simulink model "Magman_LQI"  (R2016b)
settings: Solver=VariableStepAuto  StartTime=0.0  StopTime=35  RelTol=1e-3
values from neighbouring files (symbols this model uses):
  A = [0 1;0 -mu/m]    [PID_script.m]    (also in fminsim.m = []; model_generation.m = [ 0 1 ; 0 0])
  a = 5.713e-09    [LQI_script.m]    (also in PID_script.m = 4.367e-09; fminsim.m = block.InputPort(3).Data; model_generation.m = 4.367e-09)
  b = 0.000324    [LQI_script.m]    (also in PID_script.m = 0.0002827; fminsim.m = block.InputPort(4).Data; model_generation.m = 0.0002827)
  C = [1 0]    [PID_script.m]    (also in model_generation.m)
  D = 0    [PID_script.m]
  h = 0.01    [LQI_script.m]    (also in PID_script.m; model_generation.m)
  K = lqi(sys,q,r,N)    [LQI_script.m]
  linpos = (x2+x3)/2    (= 0.06255)    [LQI_script.m]
  m = 56.3/1000    (= 0.0563)    [LQI_script.m]    (also in PID_script.m; model_generation.m)
  mu = 0.04    [LQI_script.m]    (also in PID_script.m)
  pos_var = 5e-09    [LQI_script.m]    (also in PID_script.m)
  R = pos_var    (= 5e-09)    [LQI_script.m]
  ref = linpos+0.007    (= 0.06955)    [LQI_script.m]
  x00 = linpos-0.013    (= 0.04955)    [LQI_script.m]    (also in PID_script.m = 0.03)
  x1 = 0.02525    [LQI_script.m]    (also in PID_script.m; fminsim.m = block.InputPort(5).Data; model_generation.m)
  x2 = 0.05    [LQI_script.m]    (also in PID_script.m; fminsim.m = block.InputPort(6).Data; model_generation.m)
  x3 = 0.0751    [LQI_script.m]    (also in PID_script.m; fminsim.m = block.InputPort(7).Data; model_generation.m)
  x4 = 0.103    [LQI_script.m]    (also in PID_script.m; fminsim.m = block.InputPort(8).Data; model_generation.m)
undefined symbols (not defined in the file or in its folder): Bkalm, Discrete, Time
libraries: ctrlSharedLib x1, dspsrcs4 x1
settings Model: Creator=Andres  LastModifiedBy=Andres

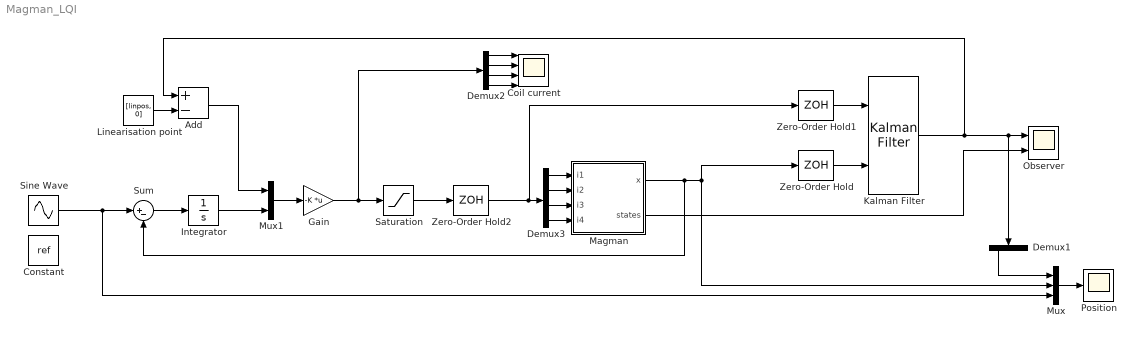
== system Magman_LQI ==
  Add : Sum  Inputs=+-
  Coil current : Scope  NumInputPorts=4
  Constant : Constant  Value=ref
  Demux1 : Demux  Outputs=2
  Demux2 : Demux
  Demux3 : Demux
  Gain : Gain  Gain=-K  Multiplication=Matrix(K*u)
  Integrator : Integrator
  Kalman Filter : ctrlSharedLib/Kalman Filter  TimeDomain=Discrete-Time  UseCurrentEstimator=off  ModelSource=LTI State-Space Variable  ModelSourceVariable=sys_d  A=A  B=Bkalm  C=C  D=D  NumberOfStates=1  NumberOfInputs=1  NumberOfOutputs=1  InitialEstimateSource=Dialog  X0=[0;x00]  P0=10  UseK=off  UseGH=off  NumberOfProcessNoiseInputs=1  G=1  TimeInvariantG=on  H=0  TimeInvariantH=on  Q=Q  TimeInvariantQ=on  R=R  TimeInvariantR=on  N=0  TimeInvariantN=on  AddInputPort=on  AddEnablePort=off  OutputEstimatedY=off  OutputP=off  Ts=-1
  Linearisation point : Constant  Value=[linpos, 0]
  Magman : Subsystem
  Mux : Mux  Inputs=3
  Mux1 : Mux  Inputs=2
  Observer : Scope  NumInputPorts=2
  Position : Scope
  Saturation : Saturate  UpperLimit=0.45  LowerLimit=0
  Sine Wave : Sin  Amplitude=0.005  Bias=x2  Frequency=0.5  SampleTime=0
  Sum : Sum  Inputs=|+-
  Zero-Order Hold : ZeroOrderHold  SampleTime=h
  Zero-Order Hold1 : ZeroOrderHold  SampleTime=h
  Zero-Order Hold2 : ZeroOrderHold  SampleTime=h
  wires:
  Zero-Order Hold2/1 -> Zero-Order Hold1/1, Demux3/1
  Magman/1(x) -> Sum/2, Mux/2, Zero-Order Hold/1
  Kalman Filter/1 -> Demux1/1, Observer/1, Add/1
  Saturation/1 -> Zero-Order Hold2/1
  Demux2/1 -> Coil current/1
  Demux2/2 -> Coil current/2
  Demux2/3 -> Coil current/3
  Demux2/4 -> Coil current/4
  Gain/1 -> Demux2/1, Saturation/1
  Mux1/1 -> Gain/1
  Integrator/1 -> Mux1/2
  Sum/1 -> Integrator/1
  Sine Wave/1 -> Mux/3, Sum/1
  Mux/1 -> Position/1
  Demux3/1 -> Magman/1(i1)
  Demux3/2 -> Magman/2(i2)
  Demux3/3 -> Magman/3(i3)
  Demux3/4 -> Magman/4(i4)
  Zero-Order Hold/1 -> Kalman Filter/2
  Zero-Order Hold1/1 -> Kalman Filter/1
  Demux1/1 -> Mux/1
  Magman/2(states) -> Observer/2
  Linearisation point/1 -> Add/2
  Add/1 -> Mux1/1

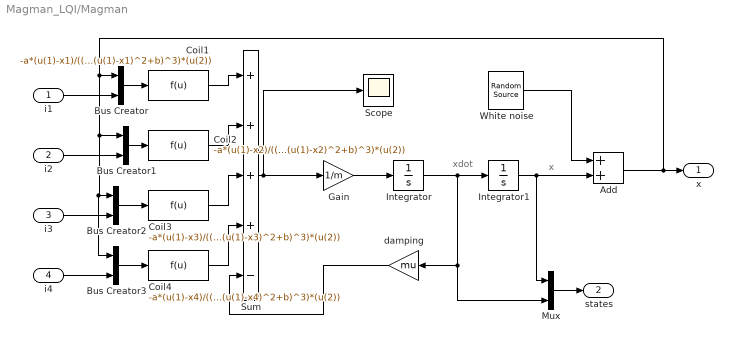
== system Magman_LQI/Magman ==
  note: x
  note: xdot
  i1 : Inport
  i2 : Inport  Port=2
  i3 : Inport  Port=3
  i4 : Inport  Port=4
  Add : Sum
  Bus Creator{,1..3} (4 alike) : BusCreator  Inputs=2
  Coil1 : Fcn  Expr=-a*(u(1)-x1)/(((u(1)-x1)^2+b)^3)*(u(2))
  Coil2 : Fcn  Expr=-a*(u(1)-x2)/(((u(1)-x2)^2+b)^3)*(u(2))
  Coil3 : Fcn  Expr=-a*(u(1)-x3)/(((u(1)-x3)^2+b)^3)*(u(2))
  Coil4 : Fcn  Expr=-a*(u(1)-x4)/(((u(1)-x4)^2+b)^3)*(u(2))
  Gain : Gain  Gain=1/m
  Integrator : Integrator  ContinuousStateAttributes='xdot'
  Integrator1 : Integrator  InitialCondition=x00  ContinuousStateAttributes='x'
  Mux : Mux  Inputs=2
  Scope : Scope
  Sum : Sum  Inputs=++++-
  White noise : dspsrcs4/Random Source  SrcType=Gaussian  NormMethod=Ziggurat  CltLength=12  MinVal=0  MaxVal=1  MeanVal=0  VarVal=2*pos_var  RepMode=Not repeatable  rawSeed=1  IsInherit=off  SampMode=Discrete  SampTime=h  SampFrame=1  DataType=Double  OutComplex=Real  OutputFrames=off
  damping : Gain  Gain=mu
  x : Outport
  states : Outport  Port=2
  wires:
  Bus Creator/1 -> Coil1/1
  Coil2/1 -> Sum/2
  i1/1 -> Bus Creator/2
  Integrator/1 -> Mux/2, damping/1, Integrator1/1
  Bus Creator2/1 -> Coil3/1
  i4/1 -> Bus Creator3/2
  Bus Creator3/1 -> Coil4/1
  Coil1/1 -> Sum/1
  i2/1 -> Bus Creator1/2
  i3/1 -> Bus Creator2/2
  Gain/1 -> Integrator/1
  Coil4/1 -> Sum/4
  Coil3/1 -> Sum/3
  Bus Creator1/1 -> Coil2/1
  damping/1 -> Sum/5
  Add/1 -> Bus Creator3/1, Bus Creator2/1, Bus Creator1/1, Bus Creator/1, x/1
  White noise/1 -> Add/1
  Sum/1 -> Gain/1, Scope/1
  Mux/1 -> states/1
  Integrator1/1 -> Mux/1, Add/2
